simulink model "questao34"  (R2020b)
settings: Solver=VariableStepAuto  StartTime=0.0  StopTime=30  RelTol=1e-3
values from neighbouring files (symbols this model uses):
  h = 1    [questao33_script.m]
  M = reshape(M,[length(M) 1])    [plotG_Gm.m]    (also in questao33_script.m = 1)
settings Model: Creator=lucas  LastModifiedBy=lucas

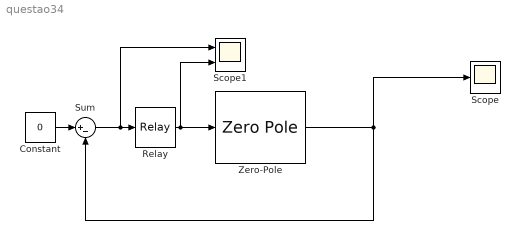
== system questao34 ==
  Constant : Constant  Value=0
  Relay : Relay  OnSwitchValue=h  OffSwitchValue=-h  OnOutputValue=M  OffOutputValue=-M  ZeroCross=off
  Scope : Scope
  Scope1 : Scope  NumInputPorts=2
  Sum : Sum  Inputs=|+-
  Zero-Pole : ZeroPole  Zeros=[]  Poles=[0 -1]
  wires:
  Relay/1 -> Scope1/2, Zero-Pole/1
  Constant/1 -> Sum/1
  Sum/1 -> Relay/1, Scope1/1
  Zero-Pole/1 -> Sum/2, Scope/1
